simulink model "Projekat_pod_c_simulink"  (R2024b)
settings: Solver=VariableStepAuto  StartTime=0.0  StopTime=10.0  RelTol=1e-3
libraries: SignalEditorBlockLib x1
settings Model: Creator=HP  LastModifiedBy=HP

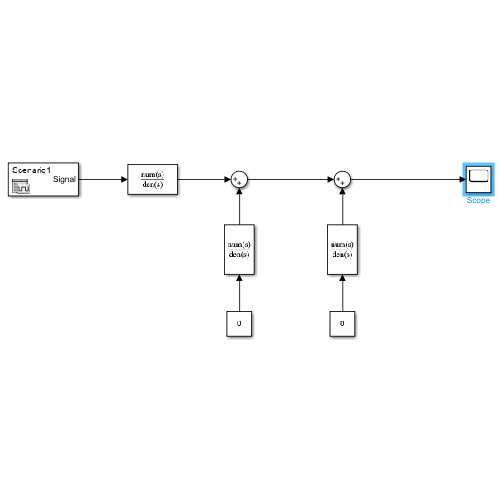
[thumbnail: Simulink's stored preview of the top-level diagram]
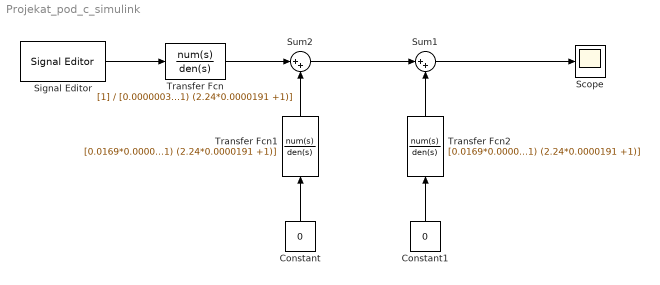
== system Projekat_pod_c_simulink ==
  Constant : Constant  Value=0
  Constant1 : Constant  Value=0
  Scope : Scope
  Signal Editor : SignalEditorBlockLib/Signal Editor  FileName=untitled.mat  ActiveScenario=Scenario1  ActiveSignal=Signal  IsBus=off  OutputBusObjectStr=Bus: BusObject  SampleTime=0  Interpolate=off  ZeroCross=off  OutputAfterFinalValue=Setting to zero  Unit=inherit  PreserveSignalName=on  ApplySigPropsToAllScenarios=on  ApplySigPropsToAllSignals=on
  Sum1 : Sum  Inputs=|++
  Sum2 : Sum  Inputs=|++
  Transfer Fcn : TransferFcn  Denominator=[0.000000382*0.0169 (2.24*0.000000382 + 0.0169*0.0000191) (2.24*0.0000191 +1)]
  Transfer Fcn1 : TransferFcn  Numerator=[0.0169*0.000000382 (2.24*0.0000191 +1)]  Denominator=[0.000000382*0.0169 (2.24*0.000000382 + 0.0169*0.0000191) (2.24*0.0000191 +1)]
  Transfer Fcn2 : TransferFcn  Numerator=[0.0169*0.000000382]  Denominator=[0.000000382*0.0169 (2.24*0.000000382 + 0.0169*0.0000191) (2.24*0.0000191 +1)]
  wires:
  Signal Editor/1 -> Transfer Fcn/1
  Constant/1 -> Transfer Fcn1/1
  Transfer Fcn/1 -> Sum2/1
  Transfer Fcn1/1 -> Sum2/2
  Sum2/1 -> Sum1/1
  Constant1/1 -> Transfer Fcn2/1
  Transfer Fcn2/1 -> Sum1/2
  Sum1/1 -> Scope/1
